simulink library "INT_EngBrk_Tst"  (R2016b)
settings: Solver=VariableStepAuto  StartTime=0.0  StopTime=10.0  RelTol=1e-3
settings Model: Creator=lenovo  LastModifiedBy=lenovo

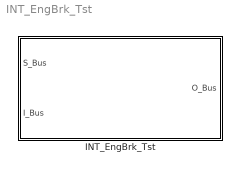
== system INT_EngBrk_Tst ==
  INT_EngBrk_Tst : Subsystem

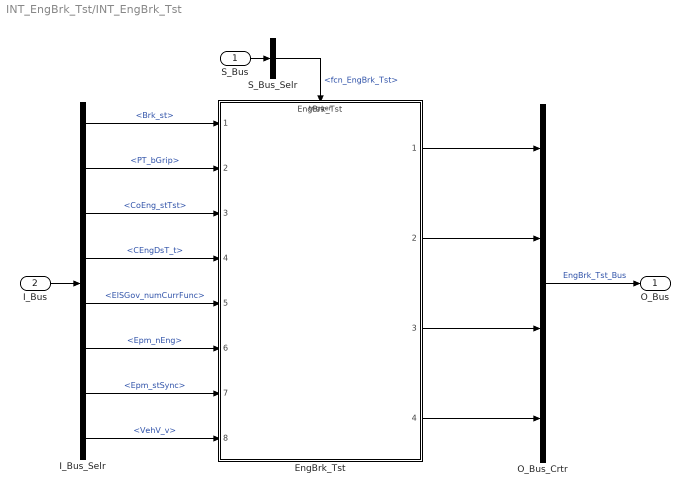
== system INT_EngBrk_Tst/INT_EngBrk_Tst ==
  S_Bus : Inport
  I_Bus : Inport  Port=2
  EngBrk_Tst : ModelReference  ModelNameDialog=EngBrk_Tst  ModelReferenceVersion=1.1  TriggerPortName=function  TriggerPortTriggerType=function-call  TriggerPortStatesWhenEnabling=held
  I_Bus_Selr : BusSelector  OutputSignals=Brk_st,PT_bGrip,CoEng_stTst,CEngDsT_t,EISGov_numCurrFunc,Epm_nEng,Epm_stSync,VehV_v
  O_Bus_Crtr : BusCreator  Inputs=4
  S_Bus_Selr : BusSelector  OutputSignals=fcn_EngBrk_Tst
  O_Bus : Outport
  wires:
  S_Bus_Selr/1 -> EngBrk_Tst/Trigger  "<fcn_EngBrk_Tst>"
  S_Bus/1 -> S_Bus_Selr/1
  I_Bus/1 -> I_Bus_Selr/1
  I_Bus_Selr/1 -> EngBrk_Tst/1  "<Brk_st>"
  I_Bus_Selr/2 -> EngBrk_Tst/2  "<PT_bGrip>"
  I_Bus_Selr/3 -> EngBrk_Tst/3  "<CoEng_stTst>"
  I_Bus_Selr/4 -> EngBrk_Tst/4  "<CEngDsT_t>"
  I_Bus_Selr/5 -> EngBrk_Tst/5  "<EISGov_numCurrFunc>"
  I_Bus_Selr/6 -> EngBrk_Tst/6  "<Epm_nEng>"
  I_Bus_Selr/7 -> EngBrk_Tst/7  "<Epm_stSync>"
  I_Bus_Selr/8 -> EngBrk_Tst/8  "<VehV_v>"
  O_Bus_Crtr/1 -> O_Bus/1  "EngBrk_Tst_Bus"
  EngBrk_Tst/1 -> O_Bus_Crtr/1
  EngBrk_Tst/2 -> O_Bus_Crtr/2
  EngBrk_Tst/3 -> O_Bus_Crtr/3
  EngBrk_Tst/4 -> O_Bus_Crtr/4
